simulink model "threeDiskOscillatorRig_Q6_experiment"  (R2020a)
settings: Solver=VariableStepAuto  StartTime=0.0  StopTime=simTime  RelTol=1e-8
values from neighbouring files (symbols this model uses):
  h = 7.56835261331    [ECP_values_final.mat]    (also in Q2-5.mat; Residual_generators.mat = 0; Residual_generatorsQ2.mat; threeDiskOscillator_ALL.m = chi2inv(1 - P_F, 1)/2)
  M = 64    [ECP_values_final.mat]    (also in GLR_function.m = 25; Q2-5.mat = 265.152560978; Residual_generatorsQ2.mat = 36; threeDiskOscillator_ALL.m = ceil(double(vpasolve([integral == P_D], [M], [0 200]))))
  mu_0 = 0    [ECP_values_final.mat]    (also in GLR.m; GLR_function.m; Q2-5.mat; Residual_generatorsQ2.mat)
  r_window = [0 0 0 0 0 0 0 0 0 0 0 0 ... (64 elements, 64x1)]    [ECP_values_final.mat]    (also in threeDiskOscillator_ALL.m = zeros(M,1); threeDiskOscillator_Q6.m = zeros(floor(M),1); threeDiskOscillator_Q8.m = zeros(floor(M),1))
  sigma_yr = 44.3946006619    [ECP_values_final.mat]    (also in Residual_generatorsQ2.mat = 0.0609223909338; threeDiskOscillator_ALL.m = sqrt(Q_yr))
  T_s = 0.004    [ECP_values_final.mat]    (also in Q2-5.mat; Residual_generators.mat; Residual_generatorsQ2.mat; threeDiskOscillator_ALL.m)
settings Model: Creator=dimpa  LastModifiedBy=Administrator
settings DataIOCC: ReturnWorkspaceOutputs=off
settings DebuggingCC: ArithmeticOperatorsInVariantConditions=warning
settings SFSimCC: SimUseLocalCustomCode=off  CustomCodeUndefinedFunction=UseInterfaceOnly
settings RTWCC: RTWUseLocalCustomCode=off

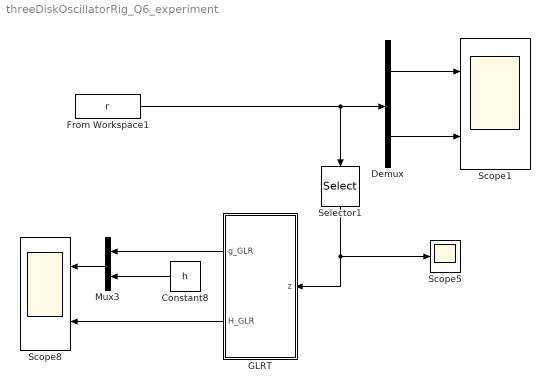
== system threeDiskOscillatorRig_Q6_experiment ==
  Constant8 : Constant  Value=h
  Demux : Demux  Outputs=2
  From Workspace1 : FromWorkspace  VariableName=r  SampleTime=T_s
  GLRT : Subsystem
  Mux3 : Mux  Inputs=2
  Scope1 : Scope  NumInputPorts=2
  Scope5 : Scope
  Scope8 : Scope  NumInputPorts=2
  Selector1 : Selector  InputPortWidth=2  IndexOptions=Index vector (dialog)  Indices=[2]  OutputSizes=1
  wires:
  From Workspace1/1 -> Selector1/1, Demux/1
  GLRT/1(g_GLR) -> Mux3/1
  GLRT/2(H_GLR) -> Scope8/2
  Constant8/1 -> Mux3/2
  Mux3/1 -> Scope8/1
  Demux/1 -> Scope1/1
  Demux/2 -> Scope1/2
  Selector1/1 -> Scope5/1, GLRT/1(z)

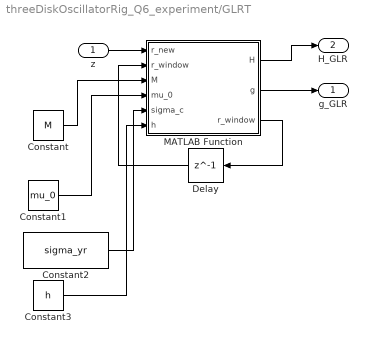
== system threeDiskOscillatorRig_Q6_experiment/GLRT ==
  z : Inport
  Constant : Constant  Value=M
  Constant1 : Constant  Value=mu_0
  Constant2 : Constant  Value=sigma_yr
  Constant3 : Constant  Value=h
  Delay : Delay  DelayLength=1  InitialCondition=r_window  SampleTime=T_s
  MATLAB Function : MATLAB Function  TreatAsAtomicUnit=on
  g_GLR : Outport  VectorParamsAs1DForOutWhenUnconnected=off
  H_GLR : Outport  Port=2  VectorParamsAs1DForOutWhenUnconnected=off
  wires:
  z/1 -> MATLAB Function/1(r_new)
  MATLAB Function/3(r_window) -> Delay/1
  MATLAB Function/2(g) -> g_GLR/1
  MATLAB Function/1(H) -> H_GLR/1
  Delay/1 -> MATLAB Function/2("r_window ")
  Constant2/1 -> MATLAB Function/5(sigma_c)
  Constant1/1 -> MATLAB Function/4(mu_0)
  Constant/1 -> MATLAB Function/3(M)
  Constant3/1 -> MATLAB Function/6(h)

== matlab function threeDiskOscillatorRig_Q6_experiment/GLRT/MATLAB Function ==
  data: r_new input; H output; r_window input; g output; r_window output; M input; mu_0 input; sigma_c input; h input
function [H, g, r_window] = GLR(r_new, r_window, M, mu_0, sigma_c, h)

%sigma = 0.36229693539067544172329302373852;
%mu_0 = 0;
%M = 265;
%h=7.5684;

r_window = [r_window(2:end); r_new];


%Using equation 7.35 from the book

%calculating g from a running window.
g = 1/(2*sigma_c^2*M)*(sum(r_window-mu_0))^2;

if (g > h)
    H = 1;
else
    H = 0;
end
